simulink model "run_sim"  (R2025a)
settings: Solver=ode5  StartTime=startTime  StopTime=stopTime  RelTol=1e-3
values from neighbouring files (symbols this model uses):
  A_max = 4    [main.m]
  alpha1 = 559.35    [main.m]
  alpha2 = 188.95    [main.m]
  beta = 379    [main.m]
  gamma0 = (-10)*deg2rad    (= -0.174532925199)    [main.m]
  k_heat_flux = 5.3697e-5    (= 5.3697e-05)    [main.m]
  L_over_D = 0.54    [main.m]
  M = 3.15    [main.m]
  Mars_mu = 4.282837e13    (= 42828370000000)    [main.m]
  Mars_omega = 7.088e-5    (= 7.088e-05)    [main.m]
  Mars_radius = 3396.2e3    (= 3396200)    [main.m]
  N = 0.5    [main.m]
  phi0 = (-21.3)*deg2rad    (= -0.371755130675)    [main.m]
  psi0 = (-2.8758)*deg2rad    (= -0.0501921786289)    [main.m]
  q_max = 13e3    (= 13000)    [main.m]
  Qdot_max = 500e3    (= 500000)    [main.m]
  r0 = (h0+Mars_radius)    (= 3521200)    [main.m]
  R_s = R_star / M_CO2    (= 188.918882072)    [main.m]
  specific_heat = 1.29    [main.m]
  stepTime = 0.01    [main.m]
  theta0 = -176.40167*deg2rad    (= -3.07878994752)    [main.m]
  V0 = 4700    [main.m]
settings Model: Creator=rafae  LastModifiedBy=rafae
settings DataIOCC: ReturnWorkspaceOutputs=off

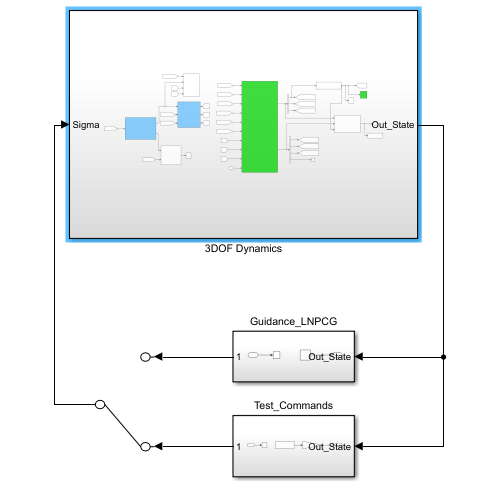
[thumbnail: Simulink's stored preview of the top-level diagram]
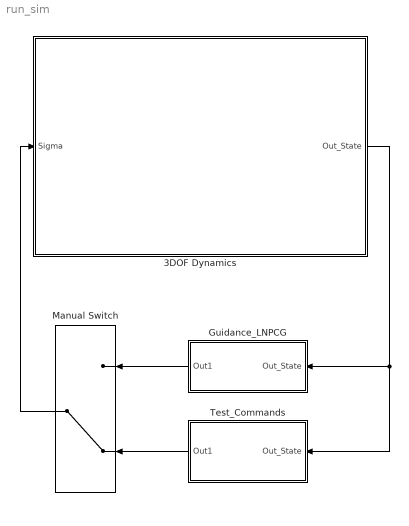
== system run_sim ==
  3DOF Dynamics : Subsystem
  Guidance_LNPCG : Subsystem
  Manual Switch : ManualSwitch  CurrentSetting=0
  Test_Commands : Subsystem
  wires:
  Guidance_LNPCG/1(Out1) -> Manual Switch/1
  Manual Switch/1 -> 3DOF Dynamics/1(Sigma)
  3DOF Dynamics/1(Out_State) -> Test_Commands/1(Out_State), Guidance_LNPCG/1(Out_State)
  Test_Commands/1(Out1) -> Manual Switch/2

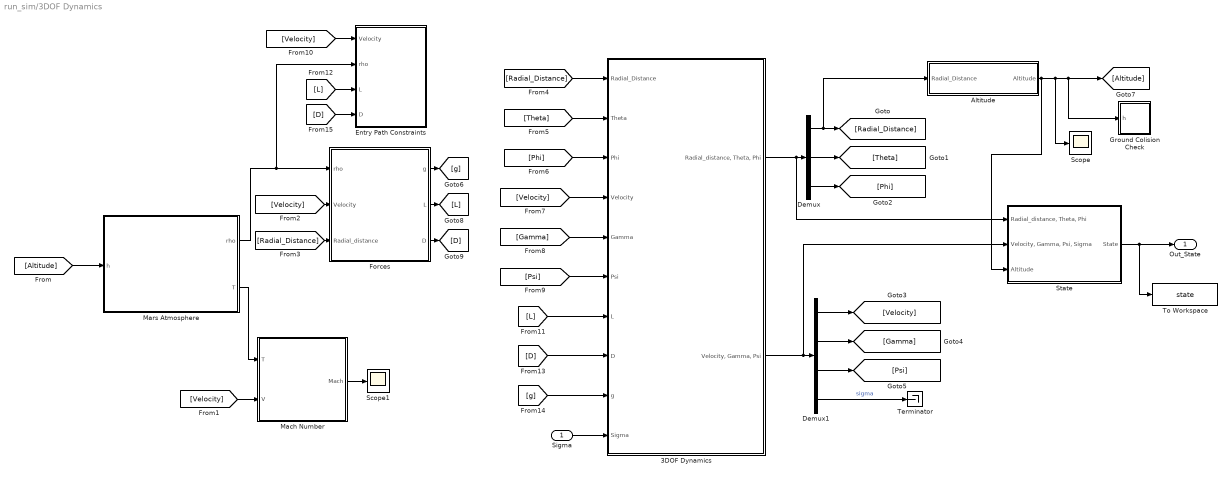
== system run_sim/3DOF Dynamics ==
  Sigma : Inport
  3DOF Dynamics : Subsystem
  Altitude : Subsystem
  Demux : Demux  Outputs=3
  Demux1 : Demux
  Entry Path Constraints : Subsystem
  Forces : Subsystem
  Ground Colision Check : Subsystem
  Mach Number : Subsystem
  Mars Atmosphere : Subsystem
  Scope : Scope
      settings: ActiveDisplayYMinimum=-15619.871180233717  ActiveDisplayYMaximum=140624.43013113708  DataLoggingVariableName=ScopeData5
  Scope1 : Scope
      settings: ActiveDisplayYMinimum=-1  ActiveDisplayYMaximum=1  DataLoggingVariableName=ScopeData15
  State : Subsystem
  Terminator : Terminator
  To Workspace : ToWorkspace  VariableName=state  SaveFormat=Structure With Time  SampleTime=-1
  Out_State : Outport
  wires:
  Mars Atmosphere/2(T) -> Mach Number/1(T)
  [Velocity] -> Mach Number/2(V)
  3DOF Dynamics/2("Velocity, Gamma, Psi") -> State/2("Velocity, Gamma, Psi, Sigma"), Demux1/1
  Demux/3 -> [Phi]
  Altitude/1(Altitude) -> State/3(Altitude), Scope/1, Ground Colision Check/1(h), [Altitude]
  Demux/1 -> Altitude/1(Radial_Distance), [Radial_Distance]
  [Radial_Distance] -> 3DOF Dynamics/1(Radial_Distance)
  [Psi] -> 3DOF Dynamics/6(Psi)
  Demux1/2 -> [Gamma]
  [Altitude] -> Mars Atmosphere/1(h)
  Demux1/1 -> [Velocity]
  State/1(State) -> Out_State/1, To Workspace/1
  Demux1/3 -> [Psi]
  [Radial_Distance] -> Forces/3(Radial_distance)
  Demux/2 -> [Theta]
  3DOF Dynamics/1("Radial_distance, Theta, Phi") -> State/1("Radial_distance, Theta, Phi"), Demux/1
  [Theta] -> 3DOF Dynamics/2(Theta)
  [Velocity] -> 3DOF Dynamics/4(Velocity)
  Mars Atmosphere/1(rho) -> Forces/1(rho), Entry Path Constraints/2(rho)
  [Gamma] -> 3DOF Dynamics/5(Gamma)
  [Velocity] -> Forces/2(Velocity)
  [Phi] -> 3DOF Dynamics/3(Phi)
  Mach Number/1(Mach) -> Scope1/1
  Sigma/1 -> 3DOF Dynamics/10(Sigma)
  Demux1/4 -> Terminator/1  "sigma"
  [Velocity] -> Entry Path Constraints/1(Velocity)
  Forces/1(g) -> [g]
  Forces/2(L) -> [L]
  Forces/3(D) -> [D]
  [L] -> Entry Path Constraints/3(L)
  [L] -> 3DOF Dynamics/7(L)
  [D] -> 3DOF Dynamics/8(D)
  [g] -> 3DOF Dynamics/9(g)
  [D] -> Entry Path Constraints/4(D)

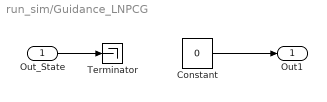
== system run_sim/Guidance_LNPCG ==
  Out_State : Inport
  Constant : Constant  Value=0
  Terminator : Terminator
  Out1 : Outport
  wires:
  Out_State/1 -> Terminator/1
  Constant/1 -> Out1/1

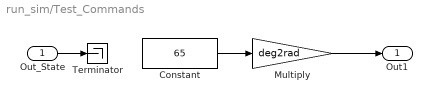
== system run_sim/Test_Commands ==
  Out_State : Inport
  Constant : Constant  Value=65
  Multiply : Gain  Gain=deg2rad
  Terminator : Terminator
  Out1 : Outport
  wires:
  Out_State/1 -> Terminator/1
  Constant/1 -> Multiply/1
  Multiply/1 -> Out1/1

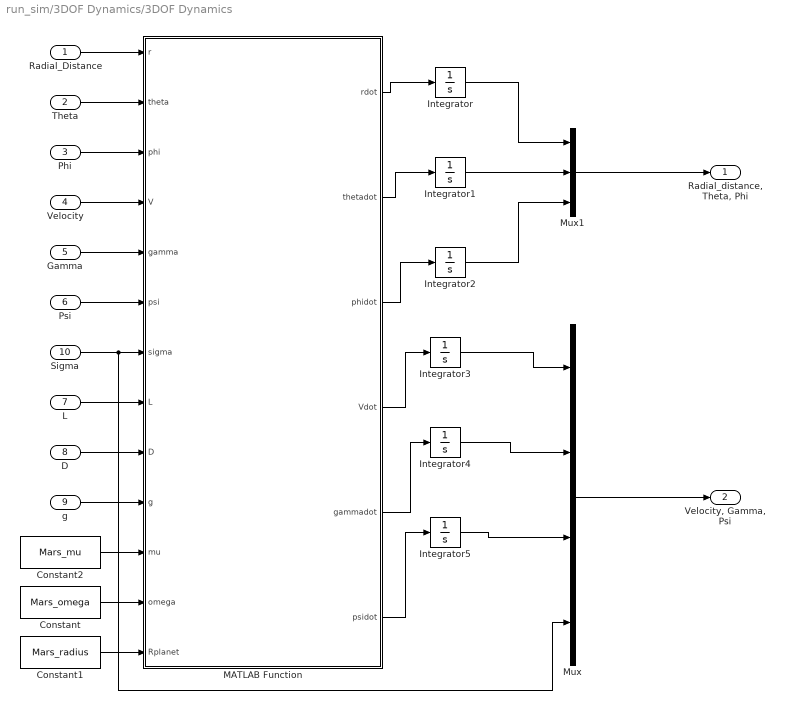
== system run_sim/3DOF Dynamics/3DOF Dynamics ==
  Radial_Distance : Inport
  Theta : Inport  Port=2
  Phi : Inport  Port=3
  Velocity : Inport  Port=4
  Gamma : Inport  Port=5
  Psi : Inport  Port=6
  L : Inport  Port=7
  D : Inport  Port=8
  g : Inport  Port=9
  Sigma : Inport  Port=10
  Constant : Constant  Value=Mars_omega
  Constant1 : Constant  Value=Mars_radius
  Constant2 : Constant  Value=Mars_mu
  Integrator : Integrator  InitialCondition=r0
  Integrator1 : Integrator  InitialCondition=theta0
  Integrator2 : Integrator  InitialCondition=phi0
  Integrator3 : Integrator  InitialCondition=V0
  Integrator4 : Integrator  InitialCondition=gamma0
  Integrator5 : Integrator  InitialCondition=psi0
  MATLAB Function : MATLAB Function  TreatAsAtomicUnit=on
  Mux : Mux
  Mux1 : Mux  Inputs=3
  "Radial_distance, Theta, Phi" : Outport
  "Velocity, Gamma, Psi" : Outport  Port=2
  wires:
  Mux1/1 -> "Radial_distance, Theta, Phi"/1
  Mux/1 -> "Velocity, Gamma, Psi"/1
  Radial_Distance/1 -> MATLAB Function/1(r)
  Theta/1 -> MATLAB Function/2(theta)
  Phi/1 -> MATLAB Function/3(phi)
  Velocity/1 -> MATLAB Function/4(V)
  Gamma/1 -> MATLAB Function/5(gamma)
  Psi/1 -> MATLAB Function/6(psi)
  Constant/1 -> MATLAB Function/12(omega)
  L/1 -> MATLAB Function/8(L)
  D/1 -> MATLAB Function/9(D)
  g/1 -> MATLAB Function/10(g)
  Constant1/1 -> MATLAB Function/13(Rplanet)
  Constant2/1 -> MATLAB Function/11(mu)
  MATLAB Function/1(rdot) -> Integrator/1
  MATLAB Function/2(thetadot) -> Integrator1/1
  MATLAB Function/3(phidot) -> Integrator2/1
  MATLAB Function/4(Vdot) -> Integrator3/1
  MATLAB Function/5(gammadot) -> Integrator4/1
  MATLAB Function/6(psidot) -> Integrator5/1
  Integrator3/1 -> Mux/1
  Integrator4/1 -> Mux/2
  Integrator5/1 -> Mux/3
  Integrator1/1 -> Mux1/2
  Integrator/1 -> Mux1/1
  Integrator2/1 -> Mux1/3
  Sigma/1 -> MATLAB Function/7(sigma), Mux/4

== system run_sim/3DOF Dynamics/Altitude ==
  Radial_Distance : Inport
  Constant : Constant  Value=Mars_radius
  Subtract : Sum  Inputs=+-
  Altitude : Outport
  wires:
  Radial_Distance/1 -> Subtract/1
  Constant/1 -> Subtract/2
  Subtract/1 -> Altitude/1

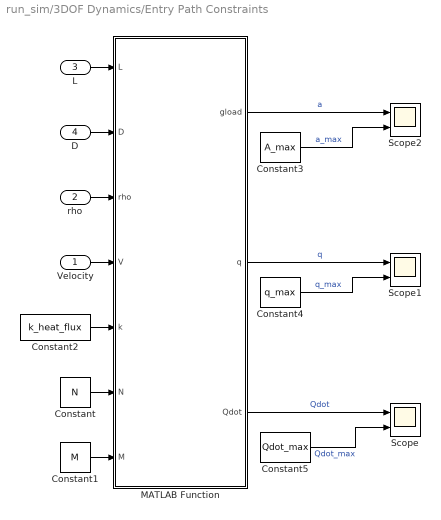
== system run_sim/3DOF Dynamics/Entry Path Constraints ==
  Velocity : Inport
  rho : Inport  Port=2
  L : Inport  Port=3
  D : Inport  Port=4
  Constant : Constant  Value=N
  Constant1 : Constant  Value=M
  Constant2 : Constant  Value=k_heat_flux
  Constant3 : Constant  Value=A_max
  Constant4 : Constant  Value=q_max
  Constant5 : Constant  Value=Qdot_max
  MATLAB Function : MATLAB Function  TreatAsAtomicUnit=on
  Scope : Scope  NumInputPorts=2
      settings: ActiveDisplayYMinimum=-58515.595205754173  ActiveDisplayYMaximum=562057.28835619485  DataLoggingVariableName=ScopeData16
  Scope1 : Scope  NumInputPorts=2
      settings: ActiveDisplayYMinimum=-1624.6031525854532  ActiveDisplayYMaximum=14624.955905842828  DataLoggingVariableName=ScopeData17
  Scope2 : Scope  NumInputPorts=2
      settings: ActiveDisplayYMinimum=-2.6567339476264884  ActiveDisplayYMaximum=23.9211833405647  DataLoggingVariableName=ScopeData18
  wires:
  Velocity/1 -> MATLAB Function/4(V)
  L/1 -> MATLAB Function/1(L)
  rho/1 -> MATLAB Function/3(rho)
  D/1 -> MATLAB Function/2(D)
  Constant/1 -> MATLAB Function/6(N)
  Constant1/1 -> MATLAB Function/7(M)
  Constant2/1 -> MATLAB Function/5(k)
  MATLAB Function/3(Qdot) -> Scope/1  "Qdot"
  MATLAB Function/2(q) -> Scope1/1  "q"
  MATLAB Function/1(gload) -> Scope2/1  "a"
  Constant3/1 -> Scope2/2  "a_max"
  Constant4/1 -> Scope1/2  "q_max"
  Constant5/1 -> Scope/2  "Qdot_max"

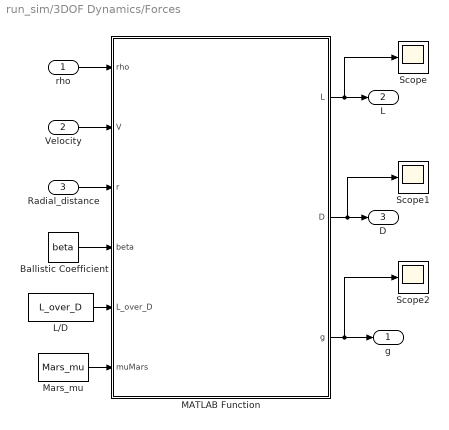
== system run_sim/3DOF Dynamics/Forces ==
  rho : Inport
  Velocity : Inport  Port=2
  Radial_distance : Inport  Port=3
  Ballistic Coefficient : Constant  Value=beta
  L/D : Constant  Value=L_over_D
  MATLAB Function : MATLAB Function  TreatAsAtomicUnit=on
  Mars_mu : Constant  Value=Mars_mu
  Scope : Scope
      settings: ActiveDisplayYMinimum=-1  ActiveDisplayYMaximum=1  DataLoggingVariableName=ScopeData2
  Scope1 : Scope
      settings: ActiveDisplayYMinimum=-1.5218684659198078  ActiveDisplayYMaximum=13.696816193278275  DataLoggingVariableName=ScopeData3
  Scope2 : Scope
      settings: DataLoggingVariableName=ScopeData4
  g : Outport
  L : Outport  Port=2
  D : Outport  Port=3
  wires:
  MATLAB Function/2(D) -> Scope1/1, D/1
  MATLAB Function/3(g) -> Scope2/1, g/1
  rho/1 -> MATLAB Function/1(rho)
  Velocity/1 -> MATLAB Function/2(V)
  Radial_distance/1 -> MATLAB Function/3(r)
  Ballistic Coefficient/1 -> MATLAB Function/4(beta)
  Mars_mu/1 -> MATLAB Function/6(muMars)
  L/D/1 -> MATLAB Function/5(L_over_D)
  MATLAB Function/1(L) -> Scope/1, L/1

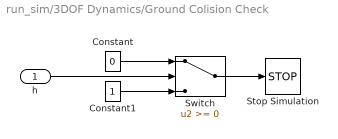
== system run_sim/3DOF Dynamics/Ground Colision Check ==
  h : Inport
  Constant : Constant  Value=0  SampleTime=stepTime
  Constant1 : Constant  SampleTime=stepTime
  Stop Simulation : Stop
  Switch : Switch  SaturateOnIntegerOverflow=off  InputSameDT=off
  wires:
  Switch/1 -> Stop Simulation/1
  Constant/1 -> Switch/1
  Constant1/1 -> Switch/3
  h/1 -> Switch/2

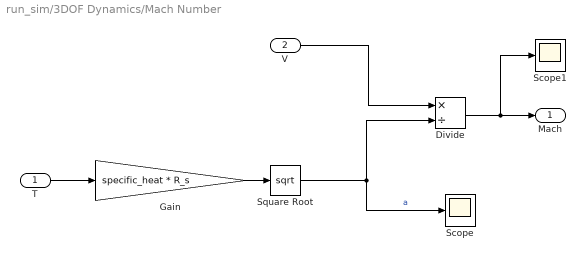
== system run_sim/3DOF Dynamics/Mach Number ==
  T : Inport
  V : Inport  Port=2
  Divide : Product  Inputs=*/
  Gain : Gain  Gain=specific_heat * R_s
  Scope : Scope
      settings: ActiveDisplayYMinimum=226.53674  ActiveDisplayYMaximum=426.53674  DataLoggingVariableName=ScopeData10
  Scope1 : Scope
      settings: ActiveDisplayYMinimum=-3.9725  ActiveDisplayYMaximum=38.23168
  Square Root : Sqrt  OutputSignalType=real
  Mach : Outport
  wires:
  Square Root/1 -> Scope/1, Divide/2  "a"
  T/1 -> Gain/1
  Gain/1 -> Square Root/1
  V/1 -> Divide/1
  Divide/1 -> Scope1/1, Mach/1

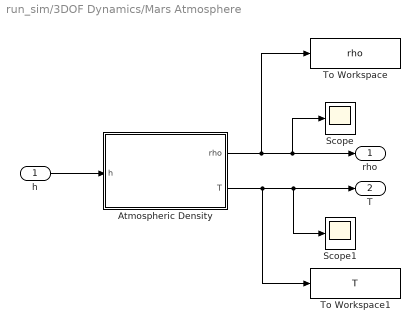
== system run_sim/3DOF Dynamics/Mars Atmosphere ==
  h : Inport
  Atmospheric Density : Subsystem
  Scope : Scope
      settings: ActiveDisplayYMinimum=-1  ActiveDisplayYMaximum=1  YLabel=kg/m^3  DataLoggingVariableName=ScopeData10
  Scope1 : Scope
      settings: ActiveDisplayYMinimum=-1  ActiveDisplayYMaximum=1  YLabel=kg/m^3
  To Workspace : ToWorkspace  VariableName=rho  SaveFormat=Structure With Time  SampleTime=-1
  To Workspace1 : ToWorkspace  VariableName=T  SaveFormat=Structure With Time  SampleTime=-1
  rho : Outport
  T : Outport  Port=2
  wires:
  h/1 -> Atmospheric Density/1(h)
  Atmospheric Density/1(rho) -> Scope/1, rho/1, To Workspace/1
  Atmospheric Density/2(T) -> To Workspace1/1, Scope1/1, T/1

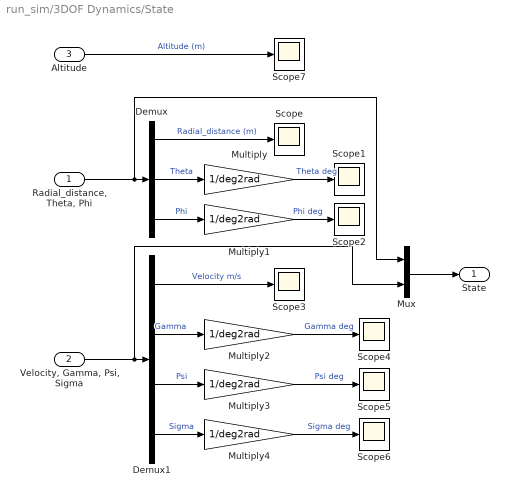
== system run_sim/3DOF Dynamics/State ==
  "Radial_distance, Theta, Phi" : Inport
  "Velocity, Gamma, Psi, Sigma" : Inport  Port=2
  Altitude : Inport  Port=3
  Demux : Demux  Outputs=3
  Demux1 : Demux
  Multiply{,1..4} (5 alike) : Gain  Gain=1/deg2rad
  Mux : Mux  Inputs=2
  Scope{,1..7} (8 alike) : Scope
      Scope settings: ActiveDisplayYMinimum=3.3811792279328117E+6  ActiveDisplayYMaximum=3.5367578635630212E+6  DataLoggingVariableName=ScopeData6
      Scope1 settings: ActiveDisplayYMinimum=-177.60933503714574  ActiveDisplayYMaximum=-171.05722499411831  DataLoggingVariableName=ScopeData7
      Scope2 settings: ActiveDisplayYMinimum=-1  ActiveDisplayYMaximum=1  DataLoggingVariableName=ScopeData8
      Scope3 settings: ActiveDisplayYMinimum=124.0759273246432  ActiveDisplayYMaximum=5246.6092246263661  DataLoggingVariableName=ScopeData9
      Scope4 settings: ActiveDisplayYMinimum=-15.21480231895317  ActiveDisplayYMaximum=3.9797883621146237  DataLoggingVariableName=ScopeData11
      Scope5 settings: ActiveDisplayYMinimum=-1  ActiveDisplayYMaximum=1  DataLoggingVariableName=ScopeData12
      Scope6 settings: ActiveDisplayYMinimum=-1  ActiveDisplayYMaximum=1  DataLoggingVariableName=ScopeData13
      Scope7 settings: ActiveDisplayYMinimum=-55007.553433071807  ActiveDisplayYMaximum=498463.37551213428  DataLoggingVariableName=ScopeData14
  State : Outport
  wires:
  "Radial_distance, Theta, Phi"/1 -> Mux/1, Demux/1
  "Velocity, Gamma, Psi, Sigma"/1 -> Mux/2, Demux1/1
  Demux/1 -> Scope/1  "Radial_distance (m)"
  Demux1/1 -> Scope3/1  "Velocity m/s"
  Demux1/2 -> Multiply2/1  "Gamma"
  Demux1/3 -> Multiply3/1  "Psi"
  Demux1/4 -> Multiply4/1  "Sigma"
  Altitude/1 -> Scope7/1  "Altitude (m)"
  Mux/1 -> State/1
  Demux/2 -> Multiply/1  "Theta"
  Multiply/1 -> Scope1/1  "Theta deg"
  Multiply1/1 -> Scope2/1  "Phi deg"
  Demux/3 -> Multiply1/1  "Phi"
  Multiply2/1 -> Scope4/1  "Gamma deg"
  Multiply3/1 -> Scope5/1  "Psi deg"
  Multiply4/1 -> Scope6/1  "Sigma deg"

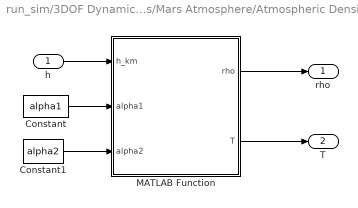
== system run_sim/3DOF Dynamics/Mars Atmosphere/Atmospheric Density ==
  h : Inport
  Constant : Constant  Value=alpha1  SampleTime=stepTime
  Constant1 : Constant  Value=alpha2  SampleTime=stepTime
  MATLAB Function : MATLAB Function  TreatAsAtomicUnit=on
  rho : Outport
  T : Outport  Port=2
  wires:
  h/1 -> MATLAB Function/1(h_km)
  Constant1/1 -> MATLAB Function/3(alpha2)
  Constant/1 -> MATLAB Function/2(alpha1)
  MATLAB Function/1(rho) -> rho/1
  MATLAB Function/2(T) -> T/1

== matlab function run_sim/3DOF Dynamics/Forces/MATLAB Function ==
  data: rho input; L output; V input; r input; beta input; L_over_D input; muMars input; D output; g output
function [L, D, g] = aero_forces(rho, V, r, beta, L_over_D, muMars)
%AERO_FORCES Computes lift, drag, and gravity acceleration for Mars entry
%
%   [L, D, g] = aero_forces(rho, V, r, beta, L_over_D, muMars)
%
% Inputs:
%   rho       - atmospheric density [kg/m^3]
%   V         - velocity magnitude [m/s]
%   r         - radial distance from Mars center [m]
%   beta      - ballistic coefficient [kg/m^2]
%   L_over_D  - lift-to-drag ratio (dimensionless)
%   muMars    - Mars gravitational parameter [m^3/s^2]
%
% Outputs:
%   L - lift acceleration [m/s^2]
%   D - drag acceleration [m/s^2]
%   g - gravitational acceleration [m/s^2]

    % Drag acceleration (Eq. above)
    D = (rho .* V.^2) ./ (2 .* beta);

    % Lift acceleration (scaled by L/D)
    L = L_over_D .* D;

    % Gravitational acceleration
    g = muMars ./ (r.^2);
end

== matlab function run_sim/3DOF Dynamics/Mars Atmosphere/Atmospheric Density/MATLAB Function ==
  data: rho output; h_km input; T output; alpha1 input; alpha2 input
function [rho, T] = mars_atmosphere(h_km,alpha1,alpha2)
%MARS_ATMOSPHERE Mars atmospheric model from Lee et al. (2024)
%
%   [rho, T] = mars_atmosphere(h_km)
%
% Inputs:
%   h_km - altitude above Martian surface [km] (can be scalar or vector)
%
% Outputs:
%   rho  - atmospheric density [kg/m^3]
%   T    - temperature [K]

    % Temperature polynomial (Eq. 15)
    T = 1.4e-13 .* h_km.^3 ...
      - 8.85e-9  .* h_km.^2 ...
      - 1.245e-3 .* h_km ...
      + 205.36;

    % Reference density rho0 (Eq. 15)
    rho0 = alpha1 ./ (alpha2 .* T);

    % Exponential atmosphere model (Eq. 14)
    rho = rho0 .* exp(-0.000105 .* h_km);
end

== matlab function run_sim/3DOF Dynamics/3DOF Dynamics/MATLAB Function ==
  data: r input; rdot output; theta input; phi input; V input; gamma input; psi input; sigma input; L input; D input; g input; mu input; omega input; Rplanet input; thetadot output; phidot output; Vdot output; gammadot output; psidot output
function [rdot, thetadot, phidot, Vdot, gammadot, psidot] = ...
    entry_dynamics(r, theta, phi, V, gamma, psi, sigma, ...
                   L, D, g, mu, omega, Rplanet)
%ENTRY_DYNAMICS Mars 3-DOF entry equations (Eqs. 1a–1f from Lee et al. 2024)
%
% Inputs:
%   r        - radial distance from planet center [m]
%   theta    - longitude [rad]
%   phi      - latitude [rad]
%   V        - velocity magnitude [m/s]
%   gamma    - flight path angle [rad]
%   psi      - azimuth / heading [rad]
%   sigma    - bank angle [rad]
%   L        - lift acceleration [m/s^2]   (input directly)
%   D        - drag acceleration [m/s^2]   (input directly)
%   g        - gravity acceleration [m/s^2] (input directly)
%   mu       - planetary gravitational parameter [m^3/s^2]
%   omega    - planetary rotation rate [rad/s]
%   Rplanet  - planetary radius [m] (not directly needed here, but included for completeness)
%
% Outputs:
%   rdot     - time derivative of radial distance [m/s]
%   thetadot - time derivative of longitude [rad/s]
%   phidot   - time derivative of latitude [rad/s]
%   Vdot     - time derivative of velocity magnitude [m/s^2]
%   gammadot - time derivative of flight path angle [rad/s]
%   psidot   - time derivative of heading angle [rad/s]

    % Equations of motion
    rdot = V * sin(gamma);

    thetadot = V * cos(gamma) * sin(psi) / (r * cos(phi));

    phidot = V * cos(gamma) * cos(psi) / r;

    Vdot = -D - g * sin(gamma) ...
           + omega^2 * r * cos(phi) * ...
             (sin(gamma) * cos(phi) - cos(gamma) * sin(phi) * cos(psi));

    gammadot = (L * cos(sigma)) / V ...
               + (V / r - g / V) * cos(gamma) ...
               + 2 * omega * cos(phi) * sin(psi) ...
               + (omega^2 * r / V) * cos(phi) * ...
                 (cos(gamma) * cos(phi) + sin(gamma) * sin(phi) * cos(psi));

    psidot = (L * sin(sigma)) / (V * cos(gamma)) ...
             + (V / r) * cos(gamma) * sin(psi) * tan(phi) ...
             + 2 * omega * (sin(phi) - tan(gamma) * cos(phi) * cos(psi)) ...
             + (omega^2 * r / (V * cos(gamma))) * sin(phi) * cos(phi) * sin(psi);
end

== matlab function run_sim/3DOF Dynamics/Entry Path Constraints/MATLAB Function ==
  data: L input; gload output; D input; rho input; V input; k input; N input; M input; q output; Qdot output
function [gload, q, Qdot] = entry_constraints(L, D, rho, V, k, N, M)
%ENTRY_CONSTRAINTS Computes load factor, dynamic pressure, and heating rate
%
% Inputs:
%   L   - lift acceleration [m/s^2]
%   D   - drag acceleration [m/s^2]
%   rho - atmospheric density [kg/m^3]
%   V   - velocity magnitude [m/s]
%   k   - heating constant
%   N   - density exponent in heating model
%   M   - velocity exponent in heating model
%
% Outputs:
%   gload   - total acceleration magnitude [m/s^2]
%   q       - dynamic pressure [Pa]
%   Qdot    - convective heating rate [W/m^2]


    % Total acceleration magnitude
    gload = sqrt(L.^2 + D.^2);

    % Dynamic pressure
    q = 0.5 .* rho .* V.^2;

    % Heating rate
    Qdot = k .* (rho.^N) .* (V.^M);
end
